simulink model "simModelHandForUSC"  (R2022a)
settings: Solver=ode4  StartTime=0.0  StopTime=4  FixedStep=0.001  RelTol=1e-3
undefined symbols (not defined in the file): sigbuilder_block
libraries: dspsigops x2
settings Model: Creator=funato  LastModifiedBy=funato

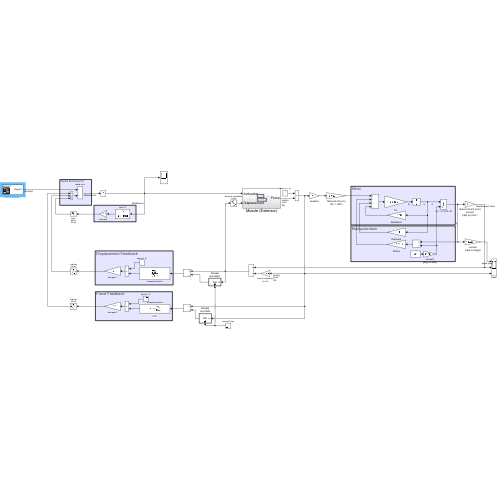
[thumbnail: Simulink's stored preview of the top-level diagram]
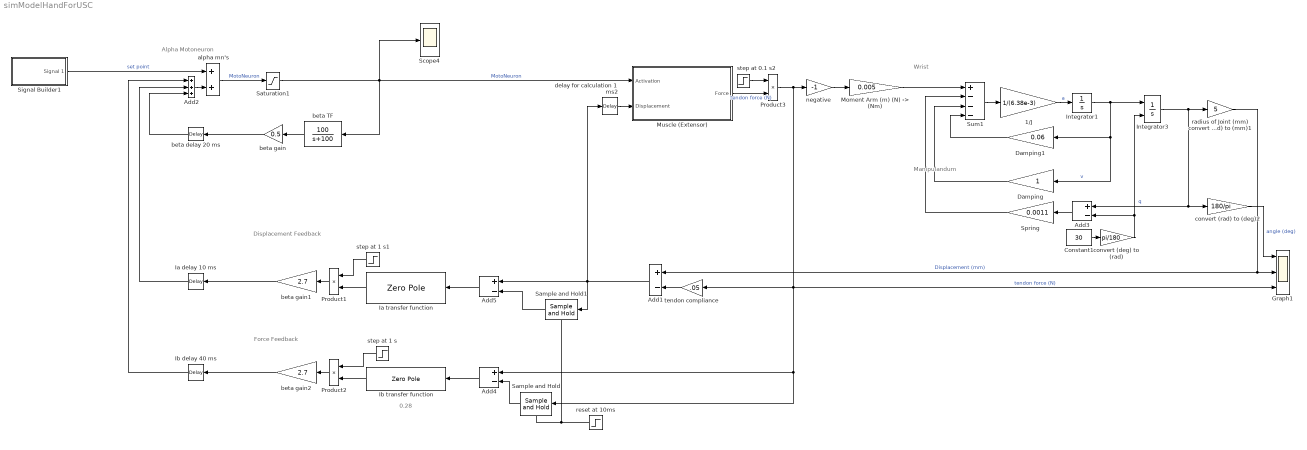
== system simModelHandForUSC ==
  note: Manipulandum
  note: Wrist
  note: 0.28
  note: Displacement Feedback
  note: Force Feedback
  note: Alpha Motoneuron
  "1/J " : Gain  Gain=1/(6.38e-3)  SaturateOnIntegerOverflow=on  OutDataTypeStr=Inherit: Same as input  ParamDataTypeStr=Inherit: Same as input
  Add{1,3..5} (4 alike) : Sum  Inputs=+-
  Add2 : Sum  Inputs=+++
  Constant1 : Constant  Value=30
  Damping : Gain  SaturateOnIntegerOverflow=on  OutDataTypeStr=Inherit: Same as input  ParamDataTypeStr=Inherit: Same as input
  Damping1 : Gain  Gain=0.06  SaturateOnIntegerOverflow=on  OutDataTypeStr=Inherit: Same as input  ParamDataTypeStr=Inherit: Same as input
  Graph1 : Scope  NumInputPorts=3
  Ia delay 10 ms : TransportDelay  DelayTime=.01
  Ia transfer function : ZeroPole  Zeros=[0; -.4; -4; -44]  Poles=[-.04; -.8; -100; -100]
  Ib delay 40 ms : TransportDelay  DelayTime=0.04
  Ib transfer function : ZeroPole  Zeros=[-.15; -1.5; -16]  Poles=[-.2; -2; -37]  Gain=[0.28]
  Integrator1 : Integrator
  Integrator3 : Integrator  InitialConditionSource=external  InitialCondition=0.5236
      settings: AttributesFormatString=q0 = %<InitialCondition> rad
  "Moment Arm (m) (N) -> (Nm)" : Gain  Gain=0.005
  Muscle (Extensor) : Subsystem
  Product1 : Product  InputSameDT=on  RndMeth=Zero  SaturateOnIntegerOverflow=on  OutDataTypeStr=Inherit: Same as first input
  Product2 : Product  InputSameDT=on  RndMeth=Zero  SaturateOnIntegerOverflow=on  OutDataTypeStr=Inherit: Same as first input
  Product3 : Product  InputSameDT=on  RndMeth=Zero  SaturateOnIntegerOverflow=on  OutDataTypeStr=Inherit: Same as first input
  Sample and Hold : dspsigops/Sample and Hold  trig=Rising edge  initCond=0  latchinput=off
  Sample and Hold1 : dspsigops/Sample and Hold  trig=Rising edge  initCond=0  latchinput=off
  Saturation1 : Saturate  UpperLimit=inf  LowerLimit=0
  Scope4 : Scope
  Signal Builder1 : Subsystem  Tag=STV Subsys  LoadFcn=sigbuilder_block('load');  StartFcn=sigbuilder_block('start');  StopFcn=sigbuilder_block('stop');  ClipboardFcn=sigbuilder_block('clipboard');  mask(Sigbuilder block){tuvar=[0:10]}
      mask help: Simulink:masks:SigbuilderBlock_MD
      mask init:
      | if ~strcmp(get_param(bdroot(gcbh),'SimulationStatus'),'stopped') tuvar = sigbuilder_block('maskInit'); end
      settings: CopyFcn=sigbuilder_block('copy');  DeleteFcn=sigbuilder_block('delete');  ModelCloseFcn=sigbuilder_block('modelClose');  PreSaveFcn=sigbuilder_block('preSave');  PauseFcn=sigbuilder_block('pause');  ContinueFcn=sigbuilder_block('continue');  NameChangeFcn=sigbuilder_block('namechange');  OpenFcn=sigbuilder_block('open',[-1017 103.714 550.286 402.429 ]);  CloseFcn=sigbuilder_block('close');
      mask Display: plot(0, 0, 100, 100,[2, 2, 32, 32, 2], [68, 8, 8, 68, 68],[32, 2], [38, 38], [32, 19, 2],[53, 60, 44], [32, 17, 17, 2],[16, 16, 31, 31]);txt = getActiveGroup(gcbh);text(2, 100, txt,'verticalAlignment', 'top');
  Spring : Gain  Gain=0.0011  SaturateOnIntegerOverflow=on  OutDataTypeStr=Inherit: Same as input  ParamDataTypeStr=Inherit: Same as input
  Sum1 : Sum  Inputs=+---  InputSameDT=on  SaturateOnIntegerOverflow=on  OutDataTypeStr=Inherit: Same as first input
  alpha mn's : Sum  InputSameDT=on  SaturateOnIntegerOverflow=on  OutDataTypeStr=Inherit: Same as first input
  beta delay 20 ms : TransportDelay  DelayTime=.02
  beta TF : TransferFcn  Numerator=[100]  Denominator=[1 100]
  beta gain : Gain  Gain=0.5  SaturateOnIntegerOverflow=on  OutDataTypeStr=Inherit: Same as input  ParamDataTypeStr=Inherit: Same as input
  beta gain1 : Gain  Gain=2.7  SaturateOnIntegerOverflow=on  OutDataTypeStr=Inherit: Same as input  ParamDataTypeStr=Inherit: Same as input
  beta gain2 : Gain  Gain=2.7  SaturateOnIntegerOverflow=on  OutDataTypeStr=Inherit: Same as input  ParamDataTypeStr=Inherit: Same as input
  convert (deg) to (rad) : Gain  Gain=pi/180
  convert (rad) to (deg)2 : Gain  Gain=180/pi
  delay for calculation 1 ms2 : TransportDelay  DelayTime=.001  InitialOutput=2.6180
  negative : Gain  Gain=-1
  radius of Joint (mm) convert (rad) to (mm)1 : Gain  Gain=5
  reset at 10ms : Step  Time=0.01  SampleTime=0.001
  step at 0.1 s2 : Step  Time=0.01  SampleTime=0.001
  step at 1 s : Step  Time=0.1  SampleTime=0.001
  step at 1 s1 : Step  Time=0.1  SampleTime=0.001
  tendon compliance : Gain  Gain=.05  SaturateOnIntegerOverflow=on  OutDataTypeStr=Inherit: Same as input  ParamDataTypeStr=Inherit: Same as input
      settings: AttributesFormatString=(mm/N)
  wires:
  "1/J "/1 -> Integrator1/1  "a"
  Sum1/1 -> "1/J "/1
  "Moment Arm (m) (N) -> (Nm)"/1 -> Sum1/1
  Add1/1 -> Sample and Hold1/1, delay for calculation 1 ms2/1, Add5/1
  Spring/1 -> Sum1/2
  Damping/1 -> Sum1/3
  Ib transfer function/1 -> Product2/2
  beta gain2/1 -> Ib delay 40 ms/1
  step at 1 s/1 -> Product2/1
  Product2/1 -> beta gain2/1
  beta gain1/1 -> Ia delay 10 ms/1
  Add2/1 -> alpha mn's/2
  beta delay 20 ms/1 -> Add2/3
  Ib delay 40 ms/1 -> Add2/1
  Saturation1/1 -> Muscle (Extensor)/1(Activation), Scope4/1, beta TF/1  "MotoNeuron"
  beta gain/1 -> beta delay 20 ms/1
  beta TF/1 -> beta gain/1
  Product1/1 -> beta gain1/1
  Ia transfer function/1 -> Product1/2
  step at 1 s1/1 -> Product1/1
  Add3/1 -> Spring/1
  Signal Builder1/1(Signal 1) -> alpha mn's/1  "set point"
  reset at 10ms/1 -> Sample and Hold/Trigger, Sample and Hold1/Trigger
  Sample and Hold/1 -> Add4/2
  Sample and Hold1/1 -> Add5/2
  delay for calculation 1 ms2/1 -> Muscle (Extensor)/2(Displacement)
  negative/1 -> "Moment Arm (m) (N) -> (Nm)"/1
  Damping1/1 -> Sum1/4
  Ia delay 10 ms/1 -> Add2/2
  Integrator1/1 -> Damping/1, Damping1/1, Integrator3/1  "v"
  convert (deg) to (rad)/1 -> Integrator3/2, Add3/2
  Product3/1 -> tendon compliance/1, Add4/1, Sample and Hold/1, Graph1/3, negative/1  "tendon force (N)"
  Integrator3/1 -> Add3/1, convert (rad) to (deg)2/1, radius of Joint (mm) convert (rad) to (mm)1/1  "q"
  Constant1/1 -> convert (deg) to (rad)/1
  radius of Joint (mm) convert (rad) to (mm)1/1 -> Graph1/2, Add1/1  "Displacement (mm)"
  convert (rad) to (deg)2/1 -> Graph1/1  "angle (deg)"
  step at 0.1 s2/1 -> Product3/1
  Muscle (Extensor)/1(Force) -> Product3/2  "tendon force (N)"
  alpha mn's/1 -> Saturation1/1  "MotoNeuron"
  Add5/1 -> Ia transfer function/1
  Add4/1 -> Ib transfer function/1
  tendon compliance/1 -> Add1/2

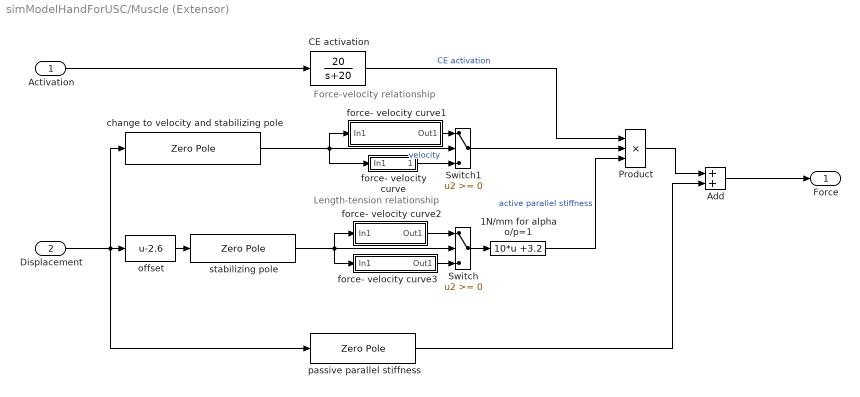
== system simModelHandForUSC/Muscle (Extensor) ==
  note: Length-tension relationship
  note: Force-velocity relationship
  Activation : Inport
  Displacement : Inport  Port=2
  1N/mm for alpha o/p=1 : Fcn  Expr=10*u +3.2
  Add : Sum
  CE activation : TransferFcn  Numerator=[20]  Denominator=[1 20]
      settings: AttributesFormatString=|
      | Low-pass Filter
      | cutoff: 20 (rad/s)=3.2Hz
  Product : Product  Inputs=3  InputSameDT=on  RndMeth=Zero  SaturateOnIntegerOverflow=on  OutDataTypeStr=Inherit: Same as first input
  Switch : Switch
  Switch1 : Switch
  change to velocity and stabilizing pole : ZeroPole  Zeros=[0]  Poles=[-500,-500]  Gain=[1500]
  force- velocity curve : Subsystem
      mask Display: disp('1/(1-u)')
  force- velocity curve1 : Subsystem
      mask Display: disp('1+.5(1-exp(-1.5u))')
  force- velocity curve2 : Subsystem
      mask Display: disp('1-exp(-.15u)')
  force- velocity curve3 : Subsystem
      mask Display: disp('-1+exp(.15u)')
  offset : Fcn  Expr=u-2.6
  passive parallel stiffness : ZeroPole  Zeros=[-25]  Poles=[-500]  Gain=[5]
      settings: AttributesFormatString=.25N/mm
  stabilizing pole : ZeroPole  Zeros=[ ]  Poles=[-500]  Gain=[500]
      settings: AttributesFormatString=|
      | Low-pass Filter
      | cutoff: %<Gain>(rad/s)
  Force : Outport
  wires:
  CE activation/1 -> Product/1  "CE activation"
  passive parallel stiffness/1 -> Add/2
  Activation/1 -> CE activation/1
  Product/1 -> Add/1
  change to velocity and stabilizing pole/1 -> force- velocity curve/1(In1), Switch1/2, force- velocity curve1/1(In1)  "velocity"
  Switch/1 -> 1N/mm for alpha o/p=1/1
  Switch1/1 -> Product/2
  stabilizing pole/1 -> force- velocity curve3/1(In1), Switch/2, force- velocity curve2/1(In1)
  force- velocity curve1/1(Out1) -> Switch1/1
  force- velocity curve/1(Out1) -> Switch1/3
  1N/mm for alpha o/p=1/1 -> Product/3  "active parallel stiffness"
  offset/1 -> stabilizing pole/1
  force- velocity curve3/1(Out1) -> Switch/3
  force- velocity curve2/1(Out1) -> Switch/1
  Displacement/1 -> passive parallel stiffness/1, change to velocity and stabilizing pole/1, offset/1
  Add/1 -> Force/1

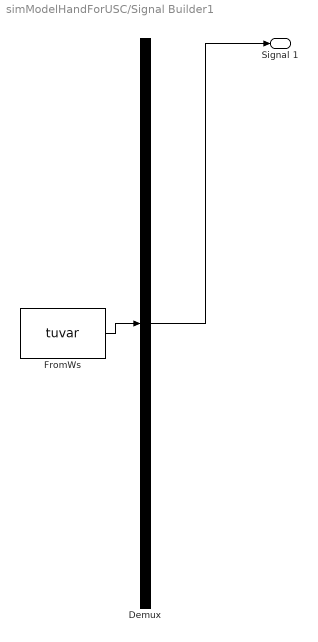
== system simModelHandForUSC/Signal Builder1 ==
  Demux : Demux  Tag=STV Demux  Outputs=1
      settings: DisplayOption=none
  FromWs : FromWorkspace  Tag=STV FromWs  VariableName=tuvar
      SigBuilderData=|
      | common.afterFinalStr = 'Extrapolate'
      | common.sampleTime = 0
      | dataSet.timeRange = [0 10]
      | dataSet.name = 'Group 1'
      | sbobj.Groups.Name = 'Group 1'
      | sbobj.Groups.Signals.Name = 'Signal 1'
      | sbobj.Groups.Signals.XData = [0 0.9 1 1.1 10]
      | sbobj.Groups.Signals.YData = [0 0 1 0 0]
  Signal 1 : Outport  Tag=STV Outport
  wires:
  Demux/1 -> Signal 1/1
  FromWs/1 -> Demux/1

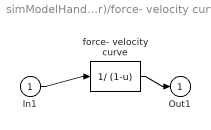
== system simModelHandForUSC/Muscle (Extensor)/force- velocity curve ==
  In1 : Inport
  force- velocity curve : Fcn  Expr=1/ (1-u)
  Out1 : Outport
  wires:
  In1/1 -> force- velocity curve/1
  force- velocity curve/1 -> Out1/1

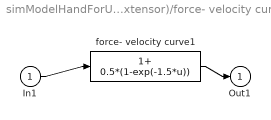
== system simModelHandForUSC/Muscle (Extensor)/force- velocity curve1 ==
  In1 : Inport
  force- velocity curve1 : Fcn  Expr=1+ 0.5*(1-exp(-1.5*u))
  Out1 : Outport
  wires:
  In1/1 -> force- velocity curve1/1
  force- velocity curve1/1 -> Out1/1

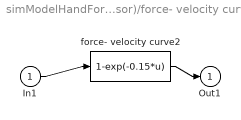
== system simModelHandForUSC/Muscle (Extensor)/force- velocity curve2 ==
  In1 : Inport
  force- velocity curve2 : Fcn  Expr=1-exp(-0.15*u)
  Out1 : Outport
  wires:
  In1/1 -> force- velocity curve2/1
  force- velocity curve2/1 -> Out1/1

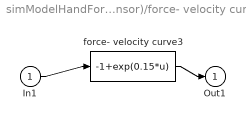
== system simModelHandForUSC/Muscle (Extensor)/force- velocity curve3 ==
  In1 : Inport
  force- velocity curve3 : Fcn  Expr=-1+exp(0.15*u)
  Out1 : Outport
  wires:
  In1/1 -> force- velocity curve3/1
  force- velocity curve3/1 -> Out1/1
